simulink model "PISim"  (R2017a)
settings: Solver=VariableStepAuto  StartTime=0.0  StopTime=60  RelTol=1e-3
values from neighbouring files (symbols this model uses):
  M = C*inv((s*eye(3)-A))*B    [PIController.m]
  Ts = 0.1    [Model_old.m]    (also in ModeloBase_OLD.m; PIController.m)
libraries: cstblocks x12, simulink x4
settings Model: Creator=davi2  LastModifiedBy=davi2

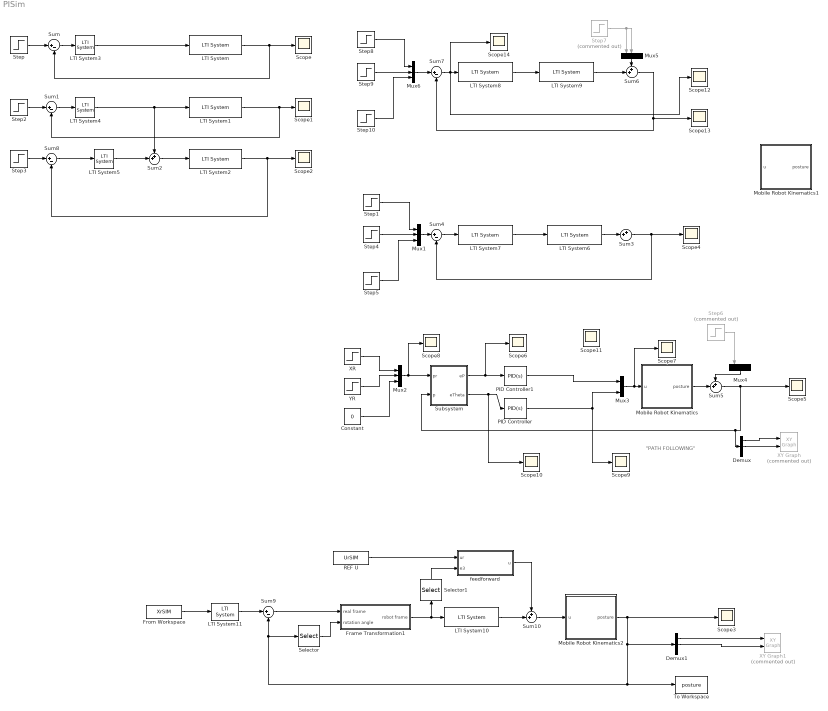
== system PISim ==
  note: "PATH FOLLOWING"
  Constant : Constant  Value=0
  Demux : Demux  Outputs=3
  Demux1 : Demux  Outputs=3
  Frame Transformation1 : Subsystem
  From Workspace : FromWorkspace  VariableName=XrSIM  SampleTime=0
  LTI System : cstblocks/LTI System  sys=M(1,1)  IC=[]
  LTI System1 : cstblocks/LTI System  sys=M(2,2)  IC=[]
  LTI System10 : cstblocks/LTI System  sys=K_PI  IC=[]
  LTI System11 : cstblocks/LTI System  sys=Kref  IC=[]
  LTI System2 : cstblocks/LTI System  sys=M(3,2)  IC=[]
  LTI System3 : cstblocks/LTI System  sys=PID  IC=[]
  LTI System4 : cstblocks/LTI System  sys=PID2  IC=[]
  LTI System5 : cstblocks/LTI System  sys=PID  IC=[]
  LTI System6 : cstblocks/LTI System  sys=M  IC=[]
  LTI System7 : cstblocks/LTI System  sys=Krga  IC=[]
  LTI System8 : cstblocks/LTI System  sys=Ksvd  IC=[]
  LTI System9 : cstblocks/LTI System  sys=M  IC=[]
  Mobile Robot Kinematics : Subsystem
  Mobile Robot Kinematics1 : Subsystem
  Mobile Robot Kinematics2 : Subsystem
  Mux{1..2,4..6} (5 alike) : Mux  Inputs=3
  Mux3 : Mux  Inputs=2
  PID Controller : simulink/Continuous/PID Controller  Controller=PID  TimeDomain=Continuous-time  SampleTime=-1  IntegratorMethod=Forward Euler  FilterMethod=Forward Euler  Form=Parallel  UseFilter=on  ControllerParametersSource=internal  P=10  I=0  D=0  N=100  InitialConditionSource=internal  InitialConditionForIntegrator=0  InitialConditionForFilter=0  ExternalReset=none  LimitOutput=off  UpperSaturationLimit=inf  LowerSaturationLimit=-inf  LinearizeAsGain=on  AntiWindupMode=none  Kb=1  TrackingMode=off  Kt=1  PParamMin=[]  PParamMax=[]  IParamMin=[]  IParamMax=[]  DParamMin=[]  DParamMax=[]  NParamMin=[]  NParamMax=[]  KbParamMin=[]  KbParamMax=[]  KtParamMin=[]  KtParamMax=[]  POutMin=[]  POutMax=[]  IOutMin=[]  IOutMax=[]  DOutMin=[]  DOutMax=[]  NOutMin=[]  NOutMax=[]  KbOutMin=[]  KbOutMax=[]  KtOutMin=[]  KtOutMax=[]  IntegratorOutMin=[]  IntegratorOutMax=[]  FilterOutMin=[]  FilterOutMax=[]  SumOutMin=[]  SumOutMax=[]  SumI1OutMin=[]  SumI1OutMax=[]  SumI2OutMin=[]  SumI2OutMax=[]  SumI3OutMin=[]  SumI3OutMax=[]  SumDOutMin=[]  SumDOutMax=[]  SaturationOutMin=[]  SaturationOutMax=[]  IntegratorContinuousStateAttributes=''  IntegratorStateMustResolveToSignalObject=off  IntegratorRTWStateStorageClass=Auto  FilterContinuousStateAttributes=''  FilterStateMustResolveToSignalObject=off  FilterRTWStateStorageClass=Auto  DifferentiatorICPrevScaledInput=0  DifferentiatorOutMin=[]  DifferentiatorOutMax=[]  InitialConditionSetting=State (most efficient)
  PID Controller1 : simulink/Continuous/PID Controller  Controller=PID  TimeDomain=Continuous-time  SampleTime=-1  IntegratorMethod=Forward Euler  FilterMethod=Forward Euler  Form=Parallel  UseFilter=on  ControllerParametersSource=internal  P=0.3  I=0  D=0  N=100  InitialConditionSource=internal  InitialConditionForIntegrator=0  InitialConditionForFilter=0  ExternalReset=none  LimitOutput=off  UpperSaturationLimit=inf  LowerSaturationLimit=-inf  LinearizeAsGain=on  AntiWindupMode=none  Kb=1  TrackingMode=off  Kt=1  PParamMin=[]  PParamMax=[]  IParamMin=[]  IParamMax=[]  DParamMin=[]  DParamMax=[]  NParamMin=[]  NParamMax=[]  KbParamMin=[]  KbParamMax=[]  KtParamMin=[]  KtParamMax=[]  POutMin=[]  POutMax=[]  IOutMin=[]  IOutMax=[]  DOutMin=[]  DOutMax=[]  NOutMin=[]  NOutMax=[]  KbOutMin=[]  KbOutMax=[]  KtOutMin=[]  KtOutMax=[]  IntegratorOutMin=[]  IntegratorOutMax=[]  FilterOutMin=[]  FilterOutMax=[]  SumOutMin=[]  SumOutMax=[]  SumI1OutMin=[]  SumI1OutMax=[]  SumI2OutMin=[]  SumI2OutMax=[]  SumI3OutMin=[]  SumI3OutMax=[]  SumDOutMin=[]  SumDOutMax=[]  SaturationOutMin=[]  SaturationOutMax=[]  IntegratorContinuousStateAttributes=''  IntegratorStateMustResolveToSignalObject=off  IntegratorRTWStateStorageClass=Auto  FilterContinuousStateAttributes=''  FilterStateMustResolveToSignalObject=off  FilterRTWStateStorageClass=Auto  DifferentiatorICPrevScaledInput=0  DifferentiatorOutMin=[]  DifferentiatorOutMax=[]  InitialConditionSetting=State (most efficient)
  REF U : FromWorkspace  VariableName=UrSIM  SampleTime=Ts  OutputAfterFinalValue=Holding final value
  Scope{,1..14} (15 alike) : Scope
  Selector : Selector  InputPortWidth=3  IndexOptions=Index vector (dialog)  Indices=3  OutputSizes=1
  Selector1 : Selector  InputPortWidth=3  IndexOptions=Index vector (dialog)  Indices=3  OutputSizes=1
  Step{,1..5,8} (7 alike) : Step  SampleTime=0
  Step10 : Step  Time=10  SampleTime=0
  Step6 : Step  Commented=on  Time=25  After=-0.4  SampleTime=0
  Step7 : Step  Commented=on  Time=15  SampleTime=0
  Step9 : Step  Time=5  SampleTime=0
  Subsystem : Subsystem
  Sum{,1,4,7..9} (6 alike) : Sum  Inputs=|+-
  Sum{2..3,5..6,10} (5 alike) : Sum  Inputs=++|
  To Workspace : ToWorkspace  VariableName=posture  SaveFormat=Timeseries  SampleTime=-1
  XR : Step  After=-2  SampleTime=0
  XY Graph : simulink/Sinks/XY Graph  Commented=on  xmin=-10  xmax=10  ymin=-10  ymax=10  st=-1
  XY Graph1 : simulink/Sinks/XY Graph  Commented=on  xmin=-1  xmax=20  ymin=-10  ymax=10  st=-1
  YR : Step  After=3  SampleTime=0
  feedforward : Subsystem
  wires:
  LTI System6/1 -> Sum3/2
  Step1/1 -> Mux1/1
  Step4/1 -> Mux1/2
  Step5/1 -> Mux1/3
  Mux1/1 -> Sum4/1
  Sum4/1 -> LTI System7/1
  Sum3/1 -> Sum4/2, Scope4/1
  Mux2/1 -> Scope8/1, Subsystem/1(pr)
  XR/1 -> Mux2/1
  YR/1 -> Mux2/2
  Constant/1 -> Mux2/3
  Subsystem/2(eTheta) -> Scope10/1, PID Controller/1
  Mux3/1 -> Scope7/1, Mobile Robot Kinematics/1(u)
  PID Controller/1 -> Mux3/2, Scope9/1
  Subsystem/1(eP) -> PID Controller1/1, Scope6/1
  LTI System7/1 -> LTI System6/1
  Demux/1 -> XY Graph/1
  Demux/2 -> XY Graph/2
  Mux4/1 -> Sum5/1
  Sum5/1 -> Demux/1, Subsystem/2(p), Scope5/1
  Mobile Robot Kinematics/1(posture) -> Sum5/2
  LTI System8/1 -> LTI System9/1
  LTI System9/1 -> Sum6/2
  Step7/1 -> Mux5/2, Mux5/1
  Mux5/1 -> Sum6/1
  Sum6/1 -> Scope13/1, Sum7/2
  Step8/1 -> Mux6/1
  Step9/1 -> Mux6/2
  Step10/1 -> Mux6/3
  Mux6/1 -> Sum7/1
  Sum7/1 -> Scope14/1, Scope12/1, LTI System8/1
  LTI System/1 -> Sum/2, Scope/1
  LTI System1/1 -> Sum1/2, Scope1/1
  LTI System2/1 -> Sum8/2, Scope2/1
  LTI System4/1 -> Sum2/1, LTI System1/1
  LTI System3/1 -> LTI System/1
  Step/1 -> Sum/1
  Sum/1 -> LTI System3/1
  Sum1/1 -> LTI System4/1
  Step2/1 -> Sum1/1
  Sum8/1 -> LTI System5/1
  Step3/1 -> Sum8/1
  LTI System5/1 -> Sum2/2
  Sum2/1 -> LTI System2/1
  Step6/1 -> Mux4/1
  PID Controller1/1 -> Mux3/1
  Sum9/1 -> Frame Transformation1/1(real frame)
  Selector/1 -> Frame Transformation1/2(rotation angle)
  Mobile Robot Kinematics2/1(posture) -> Selector/1, Sum9/2, To Workspace/1, Demux1/1, Scope3/1
  Demux1/1 -> XY Graph1/1
  Demux1/2 -> XY Graph1/2
  Frame Transformation1/1(robot frame) -> Selector1/1, LTI System10/1
  LTI System11/1 -> Sum9/1
  From Workspace/1 -> LTI System11/1
  REF U/1 -> feedforward/1(ur)
  Selector1/1 -> feedforward/2(e3)
  feedforward/1(u) -> Sum10/1
  LTI System10/1 -> Sum10/2
  Sum10/1 -> Mobile Robot Kinematics2/1(u)

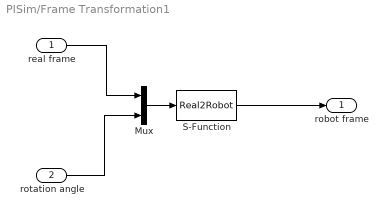
== system PISim/Frame Transformation1 ==
  real frame : Inport
  rotation angle : Inport  Port=2
  Mux : Mux  Inputs=2
  S-Function : S-Function  FunctionName=Real2Robot  Parameters=Ts  SFunctionDeploymentMode=off  EnableBusSupport=off
  robot frame : Outport
  wires:
  real frame/1 -> Mux/1
  rotation angle/1 -> Mux/2
  Mux/1 -> S-Function/1
  S-Function/1 -> robot frame/1

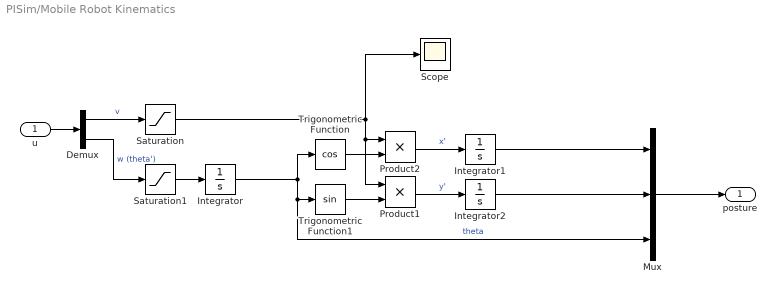
== system PISim/Mobile Robot Kinematics ==
  u : Inport
  Demux : Demux  Outputs=2
  Integrator : Integrator
  Integrator1 : Integrator
  Integrator2 : Integrator
  Mux : Mux  Inputs=3
  Product1 : Product
  Product2 : Product
  Saturation : Saturate  UpperLimit=1  LowerLimit=-1
  Saturation1 : Saturate  UpperLimit=1  LowerLimit=-1
  Scope : Scope
  Trigonometric Function : Trigonometry  Operator=cos
  Trigonometric Function1 : Trigonometry
  posture : Outport
  wires:
  u/1 -> Demux/1
  Trigonometric Function/1 -> Product2/2
  Trigonometric Function1/1 -> Product1/2
  Mux/1 -> posture/1
  Integrator/1 -> Mux/3, Trigonometric Function1/1, Trigonometric Function/1  "theta"
  Product1/1 -> Integrator2/1  "y'"
  Product2/1 -> Integrator1/1  "x'"
  Integrator1/1 -> Mux/1
  Integrator2/1 -> Mux/2
  Demux/1 -> Saturation/1  "v"
  Saturation/1 -> Scope/1, Product1/1, Product2/1
  Saturation1/1 -> Integrator/1
  Demux/2 -> Saturation1/1  "w (theta')"

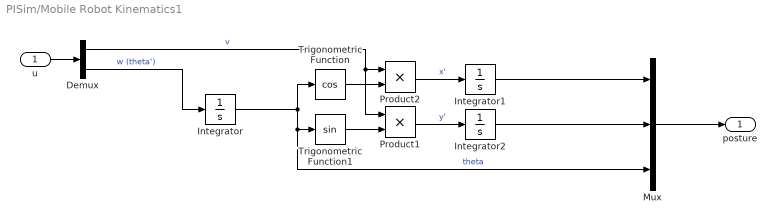
== system PISim/Mobile Robot Kinematics1 ==
  u : Inport
  Demux : Demux  Outputs=2
  Integrator : Integrator
  Integrator1 : Integrator
  Integrator2 : Integrator
  Mux : Mux  Inputs=3
  Product1 : Product
  Product2 : Product
  Trigonometric Function : Trigonometry  Operator=cos
  Trigonometric Function1 : Trigonometry
  posture : Outport
  wires:
  u/1 -> Demux/1
  Demux/2 -> Integrator/1  "w (theta')"
  Trigonometric Function/1 -> Product2/2
  Demux/1 -> Product1/1, Product2/1  "v"
  Trigonometric Function1/1 -> Product1/2
  Mux/1 -> posture/1
  Integrator/1 -> Mux/3, Trigonometric Function1/1, Trigonometric Function/1  "theta"
  Product1/1 -> Integrator2/1  "y'"
  Product2/1 -> Integrator1/1  "x'"
  Integrator1/1 -> Mux/1
  Integrator2/1 -> Mux/2

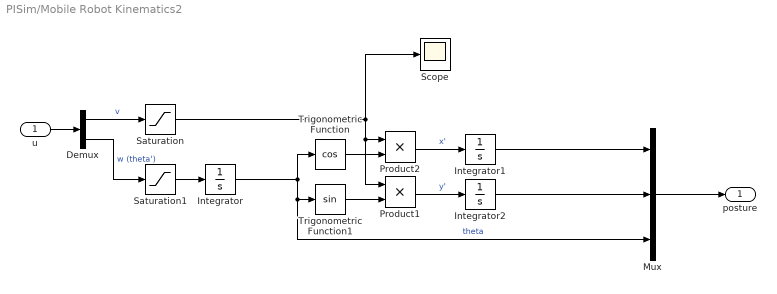
== system PISim/Mobile Robot Kinematics2 ==
  u : Inport
  Demux : Demux  Outputs=2
  Integrator : Integrator
  Integrator1 : Integrator
  Integrator2 : Integrator
  Mux : Mux  Inputs=3
  Product1 : Product
  Product2 : Product
  Saturation : Saturate  UpperLimit=1  LowerLimit=-1
  Saturation1 : Saturate  UpperLimit=1  LowerLimit=-1
  Scope : Scope
  Trigonometric Function : Trigonometry  Operator=cos
  Trigonometric Function1 : Trigonometry
  posture : Outport
  wires:
  u/1 -> Demux/1
  Trigonometric Function/1 -> Product2/2
  Trigonometric Function1/1 -> Product1/2
  Mux/1 -> posture/1
  Integrator/1 -> Mux/3, Trigonometric Function1/1, Trigonometric Function/1  "theta"
  Product1/1 -> Integrator2/1  "y'"
  Product2/1 -> Integrator1/1  "x'"
  Integrator1/1 -> Mux/1
  Integrator2/1 -> Mux/2
  Demux/1 -> Saturation/1  "v"
  Saturation/1 -> Scope/1, Product1/1, Product2/1
  Saturation1/1 -> Integrator/1
  Demux/2 -> Saturation1/1  "w (theta')"

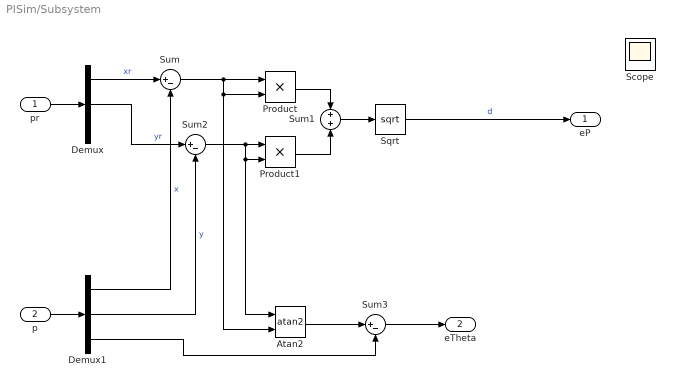
== system PISim/Subsystem ==
  pr : Inport
  p : Inport  Port=2
  Atan2 : Trigonometry  Operator=atan2
  Demux : Demux  Outputs=3
  Demux1 : Demux  Outputs=3
  Product : Product
  Product1 : Product
  Scope : Scope
  Sqrt : Sqrt  SaturateOnIntegerOverflow=on
  Sum : Sum  Inputs=|+-
  Sum1 : Sum
  Sum2 : Sum  Inputs=|+-
  Sum3 : Sum  Inputs=|+-
  eP : Outport
  eTheta : Outport  Port=2
  wires:
  p/1 -> Demux1/1
  pr/1 -> Demux/1
  Demux1/1 -> Sum/2  "x"
  Product/1 -> Sum1/1
  Demux/2 -> Sum2/1  "yr"
  Demux1/2 -> Sum2/2  "y"
  Product1/1 -> Sum1/2
  Sum1/1 -> Sqrt/1
  Demux/1 -> Sum/1  "xr"
  Sum/1 -> Product/1, Atan2/2, Product/2
  Atan2/1 -> Sum3/1
  Demux1/3 -> Sum3/2
  Sum3/1 -> eTheta/1
  Sqrt/1 -> eP/1  "d"
  Sum2/1 -> Atan2/1, Product1/2, Product1/1

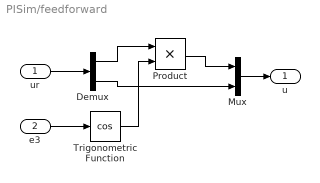
== system PISim/feedforward ==
  ur : Inport
  e3 : Inport  Port=2
  Demux : Demux  Outputs=2
  Mux : Mux  Inputs=2
  Product : Product
  Trigonometric Function : Trigonometry  Operator=cos
  u : Outport
  wires:
  e3/1 -> Trigonometric Function/1
  ur/1 -> Demux/1
  Demux/1 -> Product/1
  Trigonometric Function/1 -> Product/2
  Product/1 -> Mux/1
  Demux/2 -> Mux/2
  Mux/1 -> u/1
